simulink model "Pitch_simulink_pid_ss"  (R2018b)
settings: Solver=VariableStepAuto  StartTime=0.0  StopTime=20  RelTol=1e-3
values from neighbouring files (symbols this model uses):
  Ap = [0,1;0,sin(beta)/Iyy*(N^2/int_resist+c)*(-2*sin(beta)-Iyy/(Iw*sin(beta)))]    [Spacecraft.m]
  beta = 63.4*pi/180    (= 1.10653874576)    [Spacecraft.m]
  Bp = [0;sin(beta)*N/(Iyy*int_resist)]    [Spacecraft.m]
  Cp = [1,0;0,1]    [Spacecraft.m]
  Dp = [0;0]    [Spacecraft.m]
  int_resist = 6    [Spacecraft.m]
  Iw = max([Iw_roll Iw_pitch Iw_yaw])    [Spacecraft.m]    (also in maneuver.m = z2(end)*Is/(4*Omega_max*cos(beta)))
  Iyy = 50000    [Spacecraft.m]
  N = 60    [Spacecraft.m]
  pitch_change_angle = 30*pi/180    (= 0.523598775598)    [Spacecraft.m]
libraries: cstblocks x1
settings Model: Creator=Lucie  LastModifiedBy=Lucie

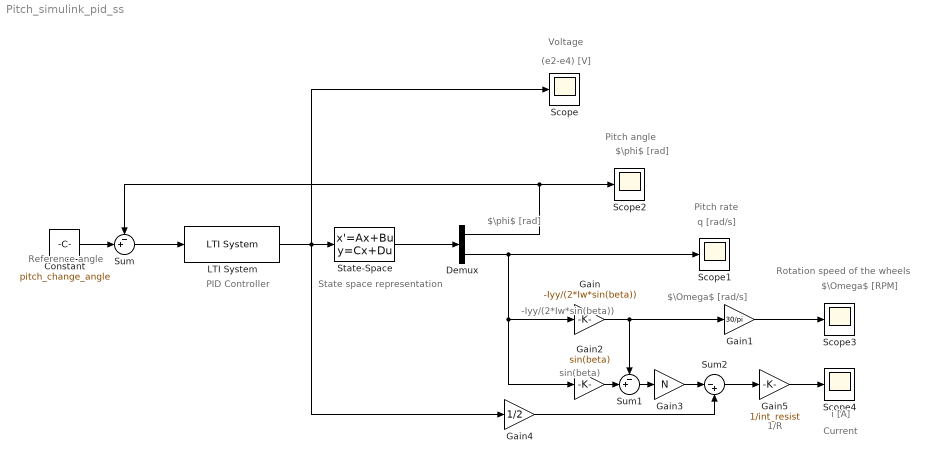
== system Pitch_simulink_pid_ss ==
  note: Current
  note: 1/R
  note: sin(beta)
  note: Rotation speed of the wheels
  note: -Iyy/(2*Iw*sin(beta))
  note: Pitch rate
  note: Pitch angle
  note: Voltage
  note: State space representation
  note: PID Controller
  note: Reference angle
  note: (e2-e4) [V]
  note: i [A]
  note: $\Omega$ [RPM]
  note: $\phi$ [rad]
  note: q [rad/s]
  note: $\Omega$ [rad/s]
  note: $\phi$ [rad]
  Constant : Constant  Value=pitch_change_angle
  Demux : Demux  Outputs=2
  Gain : Gain  Gain=-Iyy/(2*Iw*sin(beta))
  Gain1 : Gain  Gain=30/pi
  Gain2 : Gain  Gain=sin(beta)
  Gain3 : Gain  Gain=N
  Gain4 : Gain  Gain=1/2
  Gain5 : Gain  Gain=1/int_resist
  LTI System : cstblocks/LTI System  sys=C  IC=[]
  Scope{,1..4} (5 alike) : Scope
  State-Space : StateSpace  A=Ap  B=Bp  C=Cp  D=Dp  InitialCondition=0
  Sum : Sum  Inputs=-+|
  Sum1 : Sum  Inputs=-+|
  Sum2 : Sum  Inputs=|-+
  wires:
  LTI System/1 -> State-Space/1, Gain4/1, Scope/1
  Sum/1 -> LTI System/1
  Gain/1 -> Sum1/1, Gain1/1
  Gain1/1 -> Scope3/1
  Gain2/1 -> Sum1/2
  Sum1/1 -> Gain3/1
  Gain3/1 -> Sum2/1
  Gain4/1 -> Sum2/2
  Sum2/1 -> Gain5/1
  Gain5/1 -> Scope4/1
  State-Space/1 -> Demux/1
  Constant/1 -> Sum/2
  Demux/1 -> Sum/1, Scope2/1
  Demux/2 -> Scope1/1, Gain/1, Gain2/1
